simulink model "PLL_2ndType_3rdOrder_model"  (R2016a)
settings: Solver=ode45  StartTime=0  StopTime=80e-6  FixedStep=100e-12  MaxStep=1e-10  RelTol=1e-6  AbsTol=1e-12
values from neighbouring files (symbols this model uses):
  C1_num = 600e-12    (= 6e-10)    [MDLL.m]    (also in PLL_2ndType_2ndOrder.m = 2e-11; PLL_2ndType_3rdOrder.m = 4e-10)
  C2_num = 16e-12    (= 1.6e-11)    [PLL_2ndType_3rdOrder.m]
  f0 = 630e6    (= 630000000)    [DPLL_2ndType_2ndOrder.m]    (also in MDLL.m = 500000000; PLL_2ndType_2ndOrder.m = 500000000; PLL_2ndType_3rdOrder.m = 800000000; test.m = 500000000)
  fref = 200e6    (= 200000000)    [MDLL.m]    (also in PLL_2ndType_2ndOrder.m = 75000000; PLL_2ndType_3rdOrder.m = 24000000)
  N_num = 10    [DPLL_2ndType_2ndOrder.m]    (also in MDLL.m = 16; PLL_2ndType_2ndOrder.m = 8; PLL_2ndType_3rdOrder.m = 56; test.m = 20)
  R1_num = 3e3    (= 3000)    [PLL_2ndType_2ndOrder.m]    (also in PLL_2ndType_3rdOrder.m = 1000)
undefined symbols (not defined in the file): Icp_num, Kv_num
libraries: simulink_extras x2, dspswit3 x1
settings Model: SimulationMode=accelerator  Creator=asus  LastModifiedBy=xzhang
settings SolverCC: ShapePreserveControl=EnableAll  ZeroCrossControl=EnableAll  ZeroCrossAlgorithm=Adaptive
settings DataIOCC: LimitDataPoints=on  SaveFormat=Array  SignalLoggingSaveFormat=ModelDataLogs
settings OptimizationCC: ExpressionDepthLimit=2147483647  EfficientMapNaN2IntZero=off  SimCompilerOptimization=on
settings DebuggingCC: UnderspecifiedInitializationDetection=Classic  MergeDetectMultiDrivingBlocksExec=none  SolverPrmCheckMsg=warning  FcnCallInpInsideContextMsg=EnableAllAsWarning  AllowSymbolicDim=off  StateNameClashWarn=warning
settings HardwareCC: ProdBitPerPointer=32  ProdLargestAtomicFloat=None  ProdIntDivRoundTo=Undefined  ProdEndianess=Unspecified  ProdWordSize=32  ProdHWDeviceType=32-bit Generic  TargetBitPerPointer=64  TargetLongLongMode=on  TargetIntDivRoundTo=Zero  TargetEndianess=LittleEndian  TargetWordSize=64  TargetHWDeviceType=MATLAB Host  ProdEqTarget=off
settings ModelReferenceCC: PropagateSignalLabelsOutOfModel=off
settings CodeAppCC: MaxIdLength=128
settings GRTTargetCC: GeneratePreprocessorConditionals=Use local settings  CombineOutputUpdateFcns=off  GRTInterface=on
settings ConfigComp: CovModelRefEnable=Off
settings ConfigurationSet: Description=SimMechanics 2G

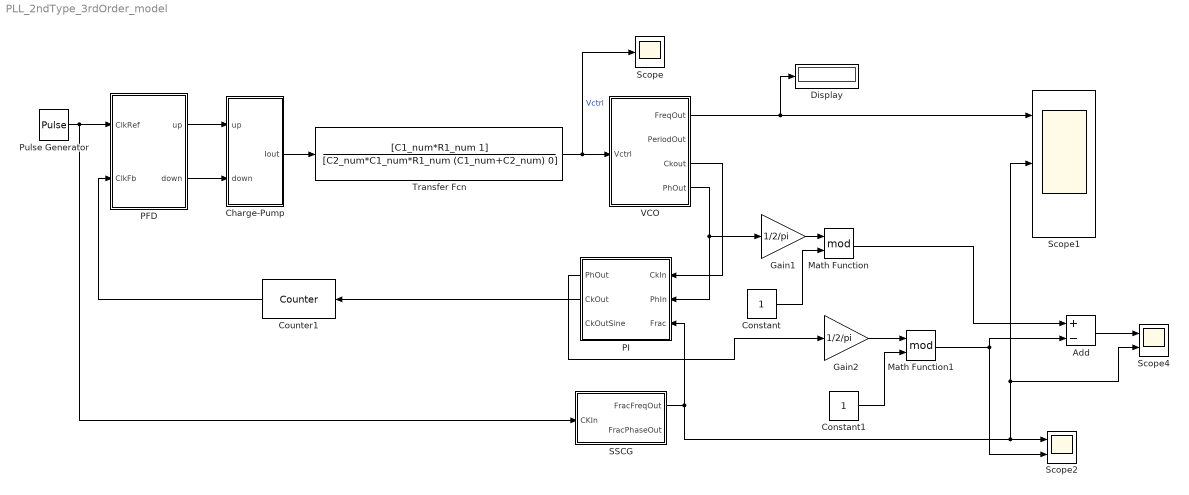
== system PLL_2ndType_3rdOrder_model ==
  Add : Sum  Inputs=+-
  Charge-Pump : Subsystem  mask{Icp=Icp_num}
      mask prompts: Icp "charge-pump current(A)"
  Constant : Constant
  Constant1 : Constant
  Counter1 : dspswit3/Counter  Direction=Up  CountEvent=Rising edge  CounterSize=User defined  MaxCount=N_num-1  InitialCount=0  Output=Hit  HitValue=N_num-1  ResetInput=off  SamplesPerFrame=1  Ts=1  CntDtype=double  HitDtype=Logical
  Display : Display
      settings: Format=short_e  Decimation=N_num
  Gain1 : Gain  Gain=1/2/pi
  Gain2 : Gain  Gain=1/2/pi
  Math Function : Math  Operator=mod  SaturateOnIntegerOverflow=on
  Math Function1 : Math  Operator=mod  SaturateOnIntegerOverflow=on
  PFD : Subsystem
  PI : Subsystem  mask{N=1}
      mask prompts: N "DivInt"
  Pulse Generator : DiscretePulseGenerator  PulseType=Time based  Period=1/fref  PulseWidth=50
  SSCG : Subsystem  mask{fsscg=30e3, Asscg=-5000, m=0, Ndiv=1, fref=fref}
      mask prompts: fsscg "SSCG Freq.(Hz)"; Asscg "SSCG AMP.(ppm)"; m "Frac Div"; Ndiv "Integer Div"; fref "RefClk Freq.(Hz)"
  Scope : Scope
  Scope1 : Scope  NumInputPorts=3
  Scope2 : Scope  NumInputPorts=2
  Scope4 : Scope  NumInputPorts=2
  Transfer Fcn : TransferFcn  Numerator=[C1_num*R1_num 1]  Denominator=[C2_num*C1_num*R1_num (C1_num+C2_num) 0]
  VCO : Subsystem  mask{f0=f0, Kvco=Kv_num}
      mask prompts: f0 "Free Running Freq.(Hz)"; Kvco "VCO Gain(Hz/V)"
  wires:
  Pulse Generator/1 -> SSCG/1(CKIn), PFD/1(ClkRef)
  PFD/1(up) -> Charge-Pump/1(up)
  PFD/2(down) -> Charge-Pump/2(down)
  Charge-Pump/1(Iout) -> Transfer Fcn/1
  Transfer Fcn/1 -> VCO/1(Vctrl), Scope/1  "Vctrl"
  VCO/1(FreqOut) -> Scope1/1, Display/1
  Counter1/1 -> PFD/2(ClkFb)
  VCO/3(Ckout) -> PI/1(CkIn)
  VCO/4(PhOut) -> PI/2(PhIn), Gain1/1
  PI/2(CkOut) -> Counter1/1
  Constant/1 -> Math Function/2
  Math Function/1 -> Add/1
  Gain1/1 -> Math Function/1
  Constant1/1 -> Math Function1/2
  Gain2/1 -> Math Function1/1
  Math Function1/1 -> Add/2, Scope2/2
  SSCG/1(FracFreqOut) -> Scope4/2, Scope1/2, Scope2/1, PI/3(Frac)
  PI/1(PhOut) -> Gain2/1
  Add/1 -> Scope4/1

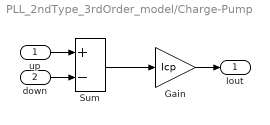
== system PLL_2ndType_3rdOrder_model/Charge-Pump ==
  up : Inport
  down : Inport  Port=2
  Gain : Gain  Gain=Icp
  Sum : Sum  Inputs=+-
  Iout : Outport
  wires:
  Sum/1 -> Gain/1
  up/1 -> Sum/1
  Gain/1 -> Iout/1
  down/1 -> Sum/2

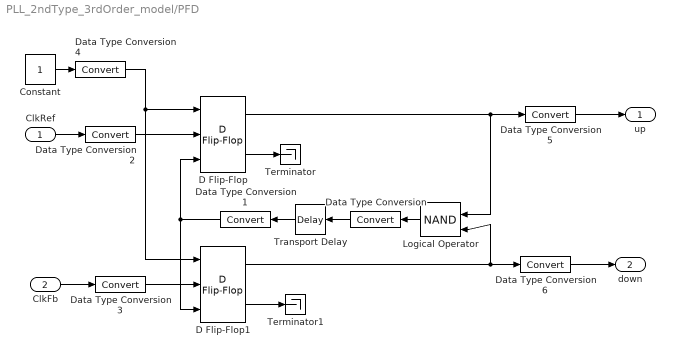
== system PLL_2ndType_3rdOrder_model/PFD ==
  ClkRef : Inport
  ClkFb : Inport  Port=2
  Constant : Constant
  D Flip-Flop : simulink_extras/Flip Flops/D Flip-Flop
  D Flip-Flop1 : simulink_extras/Flip Flops/D Flip-Flop
  Data Type Conversion{,1..6} (7 alike) : DataTypeConversion
  Logical Operator : Logic  Operator=NAND  IconShape=distinctive  AllPortsSameDT=off  OutDataTypeStr=boolean
  Terminator : Terminator
  Terminator1 : Terminator
  Transport Delay : TransportDelay  DelayTime=200e-12  BufferSize=2048
  up : Outport
  down : Outport  Port=2
  wires:
  D Flip-Flop/1 -> Logical Operator/1, Data Type Conversion5/1
  D Flip-Flop1/1 -> Logical Operator/2, Data Type Conversion6/1
  Constant/1 -> Data Type Conversion4/1
  ClkRef/1 -> Data Type Conversion2/1
  ClkFb/1 -> Data Type Conversion3/1
  Data Type Conversion/1 -> Transport Delay/1
  Transport Delay/1 -> Data Type Conversion1/1
  Logical Operator/1 -> Data Type Conversion/1
  Data Type Conversion1/1 -> D Flip-Flop1/3, D Flip-Flop/3
  D Flip-Flop/2 -> Terminator/1
  D Flip-Flop1/2 -> Terminator1/1
  Data Type Conversion2/1 -> D Flip-Flop/2
  Data Type Conversion3/1 -> D Flip-Flop1/2
  Data Type Conversion4/1 -> D Flip-Flop/1, D Flip-Flop1/1
  Data Type Conversion5/1 -> up/1
  Data Type Conversion6/1 -> down/1

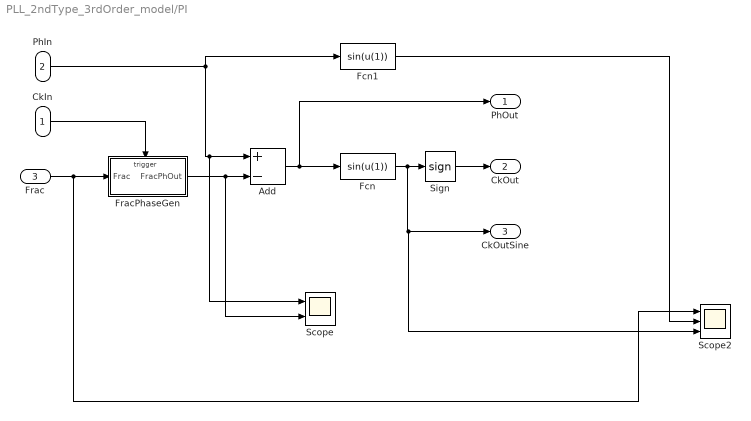
== system PLL_2ndType_3rdOrder_model/PI ==
  CkIn : Inport
  PhIn : Inport  Port=2
  Frac : Inport  Port=3
  Add : Sum  Inputs=+-
  Fcn : Fcn  Expr=sin(u(1))
  Fcn1 : Fcn  Expr=sin(u(1))
  FracPhaseGen : Subsystem  mask{N=N}
      mask prompts: N "DivInt"
  Scope : Scope  NumInputPorts=2
  Scope2 : Scope  NumInputPorts=3
  Sign : Signum
  PhOut : Outport
  CkOut : Outport  Port=2
  CkOutSine : Outport  Port=3
  wires:
  Fcn/1 -> Scope2/3, CkOutSine/1, Sign/1
  Add/1 -> PhOut/1, Fcn/1
  PhIn/1 -> Fcn1/1, Scope/1, Add/1
  CkIn/1 -> FracPhaseGen/Trigger
  Sign/1 -> CkOut/1
  FracPhaseGen/1(FracPhOut) -> Scope/2, Add/2
  Frac/1 -> Scope2/1, FracPhaseGen/1(Frac)
  Fcn1/1 -> Scope2/2

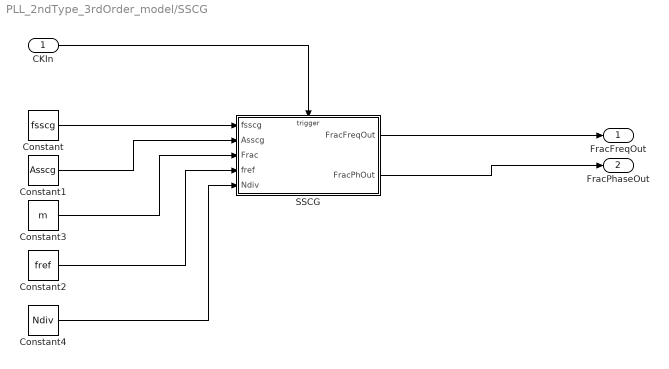
== system PLL_2ndType_3rdOrder_model/SSCG ==
  CKIn : Inport
  Constant : Constant  Value=fsscg
  Constant1 : Constant  Value=Asscg
  Constant2 : Constant  Value=fref
  Constant3 : Constant  Value=m
  Constant4 : Constant  Value=Ndiv
  SSCG : Subsystem
  FracFreqOut : Outport
  FracPhaseOut : Outport  Port=2
  wires:
  Constant/1 -> SSCG/1(fsscg)
  Constant1/1 -> SSCG/2(Asscg)
  Constant3/1 -> SSCG/3(Frac)
  CKIn/1 -> SSCG/Trigger
  Constant2/1 -> SSCG/4(fref)
  SSCG/1(FracFreqOut) -> FracFreqOut/1
  SSCG/2(FracPhOut) -> FracPhaseOut/1
  Constant4/1 -> SSCG/5(Ndiv)

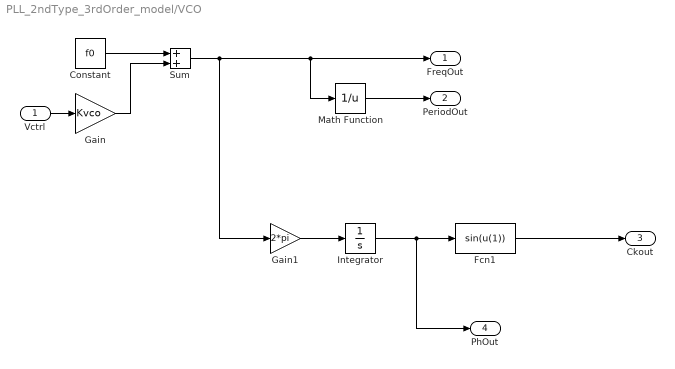
== system PLL_2ndType_3rdOrder_model/VCO ==
  Vctrl : Inport
  Constant : Constant  Value=f0
  Fcn1 : Fcn  Expr=sin(u(1))
  Gain : Gain  Gain=Kvco
  Gain1 : Gain  Gain=2*pi
  Integrator : Integrator
  Math Function : Math  Operator=reciprocal  SaturateOnIntegerOverflow=on
  Sum : Sum
  FreqOut : Outport
  PeriodOut : Outport  Port=2
  Ckout : Outport  Port=3
  PhOut : Outport  Port=4
  wires:
  Constant/1 -> Sum/1
  Gain/1 -> Sum/2
  Sum/1 -> Gain1/1, FreqOut/1, Math Function/1
  Vctrl/1 -> Gain/1
  Fcn1/1 -> Ckout/1
  Integrator/1 -> PhOut/1, Fcn1/1
  Gain1/1 -> Integrator/1
  Math Function/1 -> PeriodOut/1

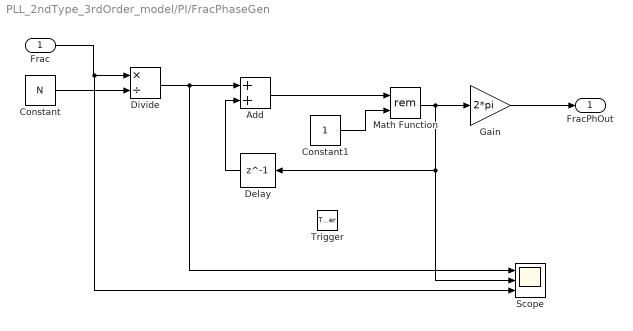
== system PLL_2ndType_3rdOrder_model/PI/FracPhaseGen ==
  Frac : Inport
  Trigger : TriggerPort  VariantControl=Variant  PortDimensions=1
  Add : Sum
  Constant : Constant  Value=N
  Constant1 : Constant
  Delay : Delay  DelayLength=1
  Divide : Product  Inputs=*/
  Gain : Gain  Gain=2*pi
  Math Function : Math  Operator=rem  SaturateOnIntegerOverflow=on
  Scope : Scope  NumInputPorts=3
  FracPhOut : Outport
  wires:
  Math Function/1 -> Scope/2, Delay/1, Gain/1
  Constant1/1 -> Math Function/2
  Add/1 -> Math Function/1
  Delay/1 -> Add/2
  Gain/1 -> FracPhOut/1
  Frac/1 -> Scope/3, Divide/1
  Constant/1 -> Divide/2
  Divide/1 -> Scope/1, Add/1

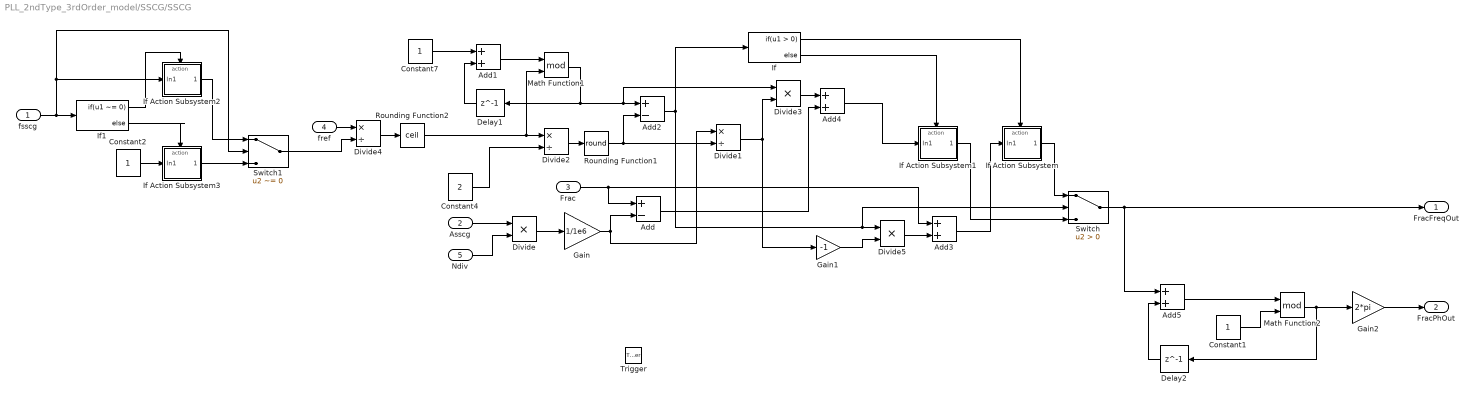
== system PLL_2ndType_3rdOrder_model/SSCG/SSCG ==
  fsscg : Inport
  Asscg : Inport  Port=2
  Frac : Inport  Port=3
  fref : Inport  Port=4
  Ndiv : Inport  Port=5
  Trigger : TriggerPort  VariantControl=Variant  PortDimensions=1
  Add : Sum  Inputs=+-
  Add1 : Sum
  Add2 : Sum  Inputs=+-
  Add3 : Sum  Inputs=2
  Add4 : Sum  Inputs=2
  Add5 : Sum
  Constant1 : Constant
  Constant2 : Constant
  Constant4 : Constant  Value=2
  Constant7 : Constant
  Delay1 : Delay  DelayLength=1
  Delay2 : Delay  DelayLength=1
  Divide : Product  Inputs=**
  Divide1 : Product  Inputs=*/
  Divide2 : Product  Inputs=*/
  Divide3 : Product
  Divide4 : Product  Inputs=*/
  Divide5 : Product
  Gain : Gain  Gain=1/1e6
  Gain1 : Gain  Gain=-1
  Gain2 : Gain  Gain=2*pi
  If : If
  If Action Subsystem : Subsystem  TreatAsAtomicUnit=on
  If Action Subsystem1 : Subsystem  TreatAsAtomicUnit=on
  If Action Subsystem2 : Subsystem  TreatAsAtomicUnit=on
  If Action Subsystem3 : Subsystem  TreatAsAtomicUnit=on
  If1 : If  IfExpression=u1 ~= 0
  Math Function1 : Math  Operator=mod  SaturateOnIntegerOverflow=on
  Math Function2 : Math  Operator=mod  SaturateOnIntegerOverflow=on
  Rounding Function1 : Rounding  Operator=round
  Rounding Function2 : Rounding  Operator=ceil
  Switch : Switch  Criteria=u2 > Threshold
  Switch1 : Switch  Criteria=u2 ~= 0
  FracFreqOut : Outport
  FracPhOut : Outport  Port=2
  wires:
  Rounding Function1/1 -> Divide1/2, Add2/2
  If Action Subsystem/1(Out1) -> Switch/1
  Math Function1/1 -> Divide3/1, Add2/1, Delay1/1
  Add1/1 -> Math Function1/1
  If/2 -> If Action Subsystem1/Action
  Constant4/1 -> Divide2/2
  Divide1/1 -> Gain1/1, Divide3/2
  If/1 -> If Action Subsystem/Action
  If Action Subsystem1/1(Out1) -> Switch/3
  Add3/1 -> If Action Subsystem/1(In1)
  Divide2/1 -> Rounding Function1/1
  Divide5/1 -> Add3/2
  Constant7/1 -> Add1/1
  Delay1/1 -> Add1/2
  Add2/1 -> Divide5/1, Switch/2, If/1
  fref/1 -> Divide4/1
  fsscg/1 -> If Action Subsystem2/1(In1), Switch1/2, If1/1
  Frac/1 -> Add3/1, Add/1
  Divide3/1 -> Add4/1
  Add4/1 -> If Action Subsystem1/1(In1)
  Gain1/1 -> Divide5/2
  Add/1 -> Add4/2
  Gain/1 -> Add/2, Divide1/1
  Math Function2/1 -> Gain2/1, Delay2/1
  Constant1/1 -> Math Function2/2
  Add5/1 -> Math Function2/1
  Delay2/1 -> Add5/2
  Switch/1 -> Add5/1, FracFreqOut/1
  Gain2/1 -> FracPhOut/1
  Divide4/1 -> Rounding Function2/1
  Constant2/1 -> If Action Subsystem3/1(In1)
  If Action Subsystem2/1(Out1) -> Switch1/1
  Switch1/1 -> Divide4/2
  If1/1 -> If Action Subsystem2/Action
  If1/2 -> If Action Subsystem3/Action
  If Action Subsystem3/1(Out1) -> Switch1/3
  Rounding Function2/1 -> Math Function1/2, Divide2/1
  Asscg/1 -> Divide/1
  Ndiv/1 -> Divide/2
  Divide/1 -> Gain/1

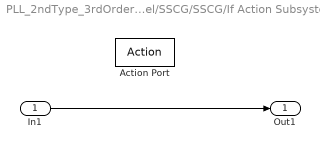
== system PLL_2ndType_3rdOrder_model/SSCG/SSCG/If Action Subsystem ==
  In1 : Inport
  Action Port : ActionPort  ActionType=then
  Out1 : Outport
  wires:
  In1/1 -> Out1/1

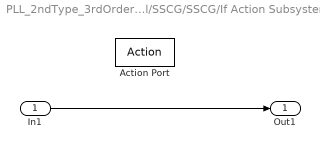
== system PLL_2ndType_3rdOrder_model/SSCG/SSCG/If Action Subsystem1 ==
  In1 : Inport
  Action Port : ActionPort  ActionType=else
  Out1 : Outport
  wires:
  In1/1 -> Out1/1

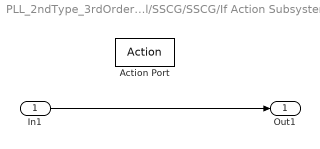
== system PLL_2ndType_3rdOrder_model/SSCG/SSCG/If Action Subsystem2 ==
  In1 : Inport
  Action Port : ActionPort  ActionType=then
  Out1 : Outport
  wires:
  In1/1 -> Out1/1

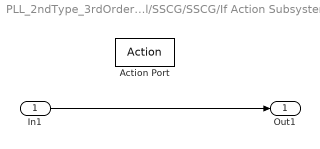
== system PLL_2ndType_3rdOrder_model/SSCG/SSCG/If Action Subsystem3 ==
  In1 : Inport
  Action Port : ActionPort  ActionType=else
  Out1 : Outport
  wires:
  In1/1 -> Out1/1
